simulink model "model"  (R2023b)
settings: Solver=VariableStepAuto  StartTime=0.0  StopTime=1  RelTol=1e-3
settings Model: Creator=diontep  LastModifiedBy=a2

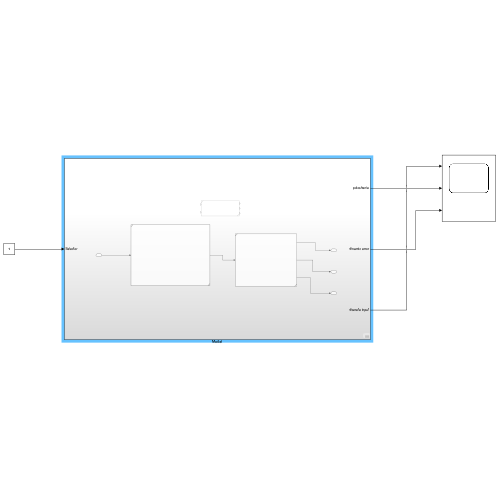
[thumbnail: Simulink's stored preview of the top-level diagram]
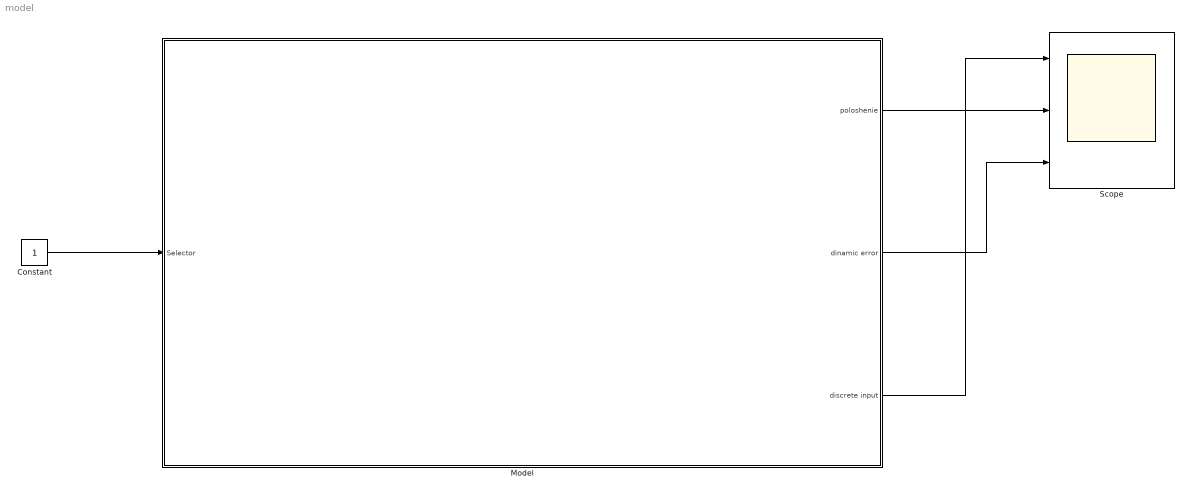
== system model ==
  Constant : Constant
  Model : Subsystem
  Scope : Scope  NumInputPorts=3
  wires:
  Model/3(discrete input) -> Scope/1
  Model/2(dinamic error) -> Scope/3
  Model/1(poloshenie) -> Scope/2
  Constant/1 -> Model/1(Selector)

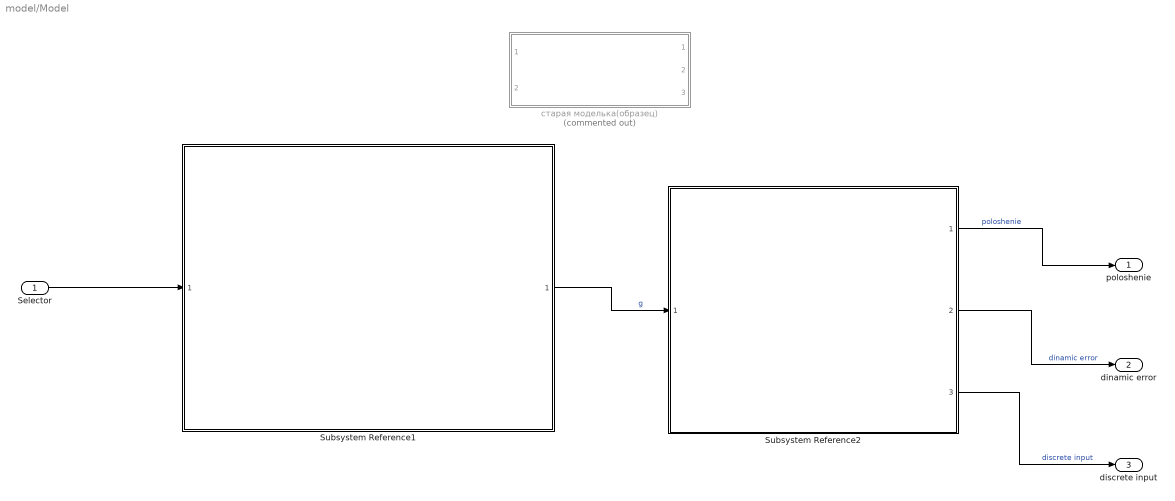
== system model/Model ==
  Selector : Inport
  Subsystem Reference1 : Subsystem  ReferencedSubsystem=testSelector  amp1=12  amp2=12  amp3=12
  Subsystem Reference2 : Subsystem  ReferencedSubsystem=ILYA_Subsystem
  старая моделька(образец) : Subsystem  Commented=on  ReferencedSubsystem=robot  K=7  T1=0.1  T2=0.05  ki=0  kp=0  kd=0
  poloshenie : Outport
  dinamic error : Outport  Port=2
  discrete input : Outport  Port=3
  wires:
  Subsystem Reference1/1 -> Subsystem Reference2/1  "g"
  Subsystem Reference2/3 -> discrete input/1  "discrete input"
  Selector/1 -> Subsystem Reference1/1
  Subsystem Reference2/1 -> poloshenie/1  "poloshenie"
  Subsystem Reference2/2 -> dinamic error/1  "dinamic error"
